simulink model "TrafficLightController_SIL_Test"  (R2024b)
settings: Solver=ode4  StartTime=0.0  StopTime=10.0  RelTol=1e-3
settings Model: Creator=adetunji  LastModifiedBy=adetunji
settings OptimizationCC: DefaultParameterBehavior=Inlined  EnhancedBackFolding=on  PassReuseOutputArgsThreshold=0  OptimizeBlockOrder=speed  DifferentSizesBufferReuse=on  OptimizationCustomize=off
settings DebuggingCC: ParameterTunabilityLossMsg=error
settings SFSimCC: MATLABDynamicMemAlloc=off
settings RTWCC: GenerateReport=on  LaunchReport=on
settings CodeAppCC: ForceParamTrailComments=on  OperatorAnnotations=on

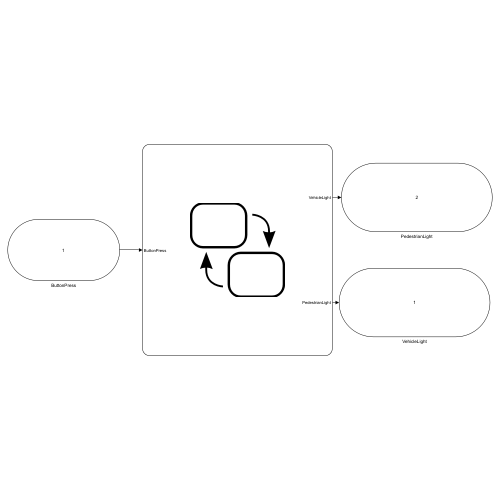
[thumbnail: Simulink's stored preview of the top-level diagram]
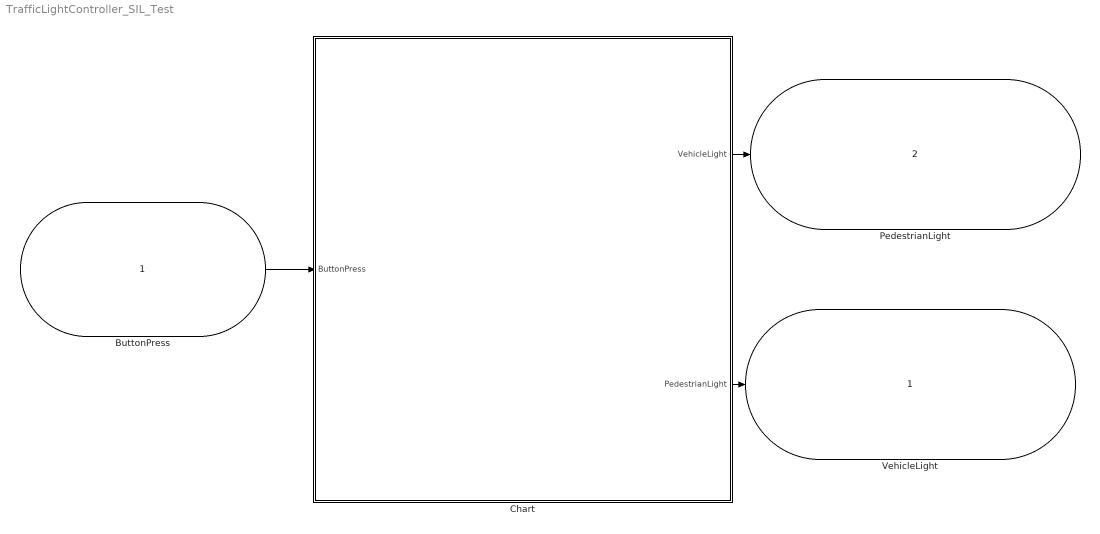
== system TrafficLightController_SIL_Test ==
  ButtonPress : Inport
  Chart : Stateflow chart  TreatAsAtomicUnit=on
  VehicleLight : Outport
  PedestrianLight : Outport  Port=2
  wires:
  ButtonPress/1 -> Chart/1(ButtonPress)
  Chart/1(VehicleLight) -> PedestrianLight/1
  Chart/2(PedestrianLight) -> VehicleLight/1

== stateflow chart TrafficLightController_SIL_Test/Chart ==
  state Crossing
    entry: VehicleLight = 1; PedestrianLight = 1;
    coder.ceval('printf', 'Traffic Light: CROSSING - Vehicle RED, Pedestrian GREEN\n');
  state Amber
    entry: VehicleLight = 2; PedestrianLight = 0;
    coder.ceval('printf', 'Traffic Light: AMBER - Vehicle AMBER, Pedestrian RED\n');
  state Idle
    entry: VehicleLight = 3; PedestrianLight = 0;
    coder.ceval('printf', 'Traffic Light: IDLE - Vehicle GREEN, Pedestrian RED\n');
  (default) -> Idle
  Amber -> Crossing : after(3,sec)
  Idle -> Amber : [ButtonPress == 1]
  Crossing -> Idle : after(15,sec)
  data: ButtonPress input size=1; VehicleLight output size=1; PedestrianLight output size=1
